simulink model "tdm_4chnl"  (R2018a)
settings: Solver=ode45  StartTime=0.0  StopTime=10  RelTol=1e-3
libraries: simulink_extras x3
settings Model: Creator=ete  LastModifiedBy=hp
settings DataIOCC: ReturnWorkspaceOutputs=on
settings OptimizationCC: LifeSpan=inf
settings DebuggingCC: SFExecutionAtInitializationDiag=none
settings HardwareCC: ProdBitPerSizeT=32  ProdBitPerPtrDiffT=32  ProdWordSize=32  ProdHWDeviceType=Specified
settings SFSimCC: SimUseLocalCustomCode=on
settings RTWCC: RTWUseLocalCustomCode=on
settings CodeAppCC: StateflowObjectComments=on

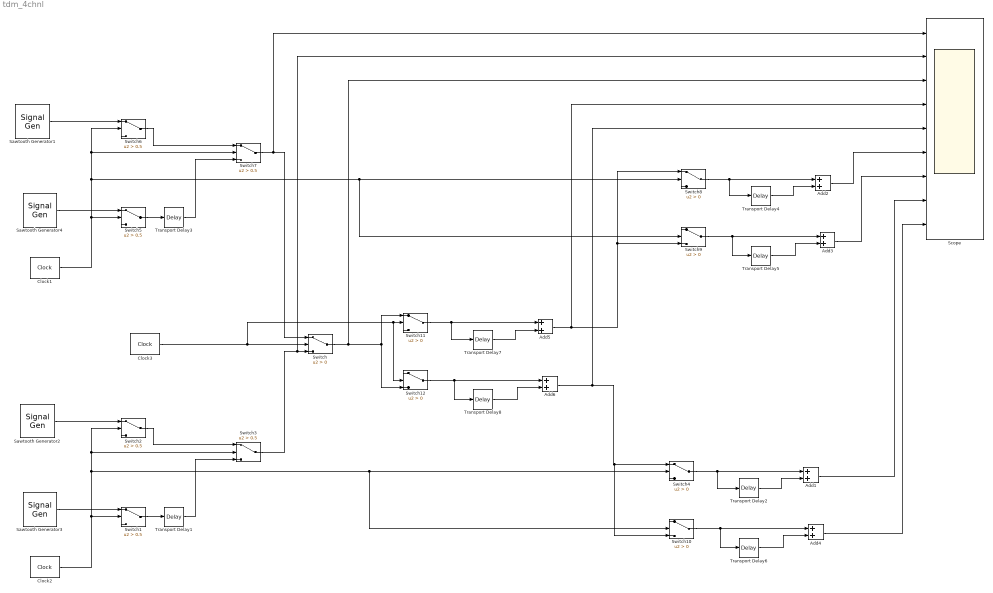
== system tdm_4chnl ==
  Add{1..6} (6 alike) : Sum
  Clock1 : simulink_extras/Flip Flops/Clock  period=2
  Clock2 : simulink_extras/Flip Flops/Clock  period=2
  Clock3 : simulink_extras/Flip Flops/Clock  period=4
  Sawtooth Generator1 : SignalGenerator  Frequency=2
  Sawtooth Generator2 : SignalGenerator  WaveForm=sawtooth  Frequency=2
  Sawtooth Generator3 : SignalGenerator  WaveForm=random  Amplitude=4  Frequency=10
  Sawtooth Generator4 : SignalGenerator  WaveForm=square  Amplitude=4  Frequency=4
  Scope : Scope  NumInputPorts=9
  Switch{,4,8..12} (7 alike) : Switch  Criteria=u2 > Threshold
  Switch{1..3,5..7} (6 alike) : Switch  Criteria=u2 > Threshold  Threshold=0.5
  Transport Delay{1..6} (6 alike) : TransportDelay
  Transport Delay7 : TransportDelay  DelayTime=2
  Transport Delay8 : TransportDelay  DelayTime=2
  wires:
  Switch8/1 -> Transport Delay4/1, Add2/1
  Clock1/1 -> Switch7/2, Switch6/2, Switch9/2, Switch8/2, Switch5/2
  Sawtooth Generator4/1 -> Switch5/1
  Switch9/1 -> Transport Delay5/1, Add3/1
  Switch6/1 -> Switch7/1
  Sawtooth Generator1/1 -> Switch6/1
  Transport Delay4/1 -> Add2/2
  Transport Delay5/1 -> Add3/2
  Switch5/1 -> Transport Delay3/1
  Transport Delay3/1 -> Switch7/3
  Transport Delay1/1 -> Switch3/3
  Switch1/1 -> Transport Delay1/1
  Sawtooth Generator2/1 -> Switch2/1
  Switch2/1 -> Switch3/1
  Sawtooth Generator3/1 -> Switch1/1
  Transport Delay6/1 -> Add4/2
  Transport Delay2/1 -> Add1/2
  Switch10/1 -> Transport Delay6/1, Add4/1
  Clock2/1 -> Switch10/2, Switch4/2, Switch3/2, Switch2/2, Switch1/2
  Switch4/1 -> Transport Delay2/1, Add1/1
  Clock3/1 -> Switch12/2, Switch11/2, Switch/2
  Switch7/1 -> Scope/1, Switch/1
  Switch3/1 -> Scope/2, Switch/3
  Transport Delay8/1 -> Add6/2
  Transport Delay7/1 -> Add5/2
  Switch12/1 -> Transport Delay8/1, Add6/1
  Switch11/1 -> Transport Delay7/1, Add5/1
  Switch/1 -> Scope/3, Switch11/1, Switch12/3
  Add5/1 -> Scope/4, Switch9/3, Switch8/1
  Add6/1 -> Scope/5, Switch10/3, Switch4/1
  Add2/1 -> Scope/6
  Add3/1 -> Scope/7
  Add1/1 -> Scope/8
  Add4/1 -> Scope/9
